simulink model "single_agent_setup"  (R2016a)
settings: Solver=VariableStepAuto  StartTime=0.0  StopTime=400  RelTol=1e-3
model workspace (MAT data in the model file):
  agent_signal = Simulink.Signal
  agent_signal.DataType = 'double'
  agent_signal.Dimensions = 2
  agent_signal.DimensionsMode = 'Variable'
  agent_signal.Complexity = 'real'
  agent_signal.SampleTime = -1
  agent_signal.SamplingMode = 'auto'
libraries: simulink x3, vrlib x3
settings Model: Creator=jcfinnerup  LastModifiedBy=jcfinnerup

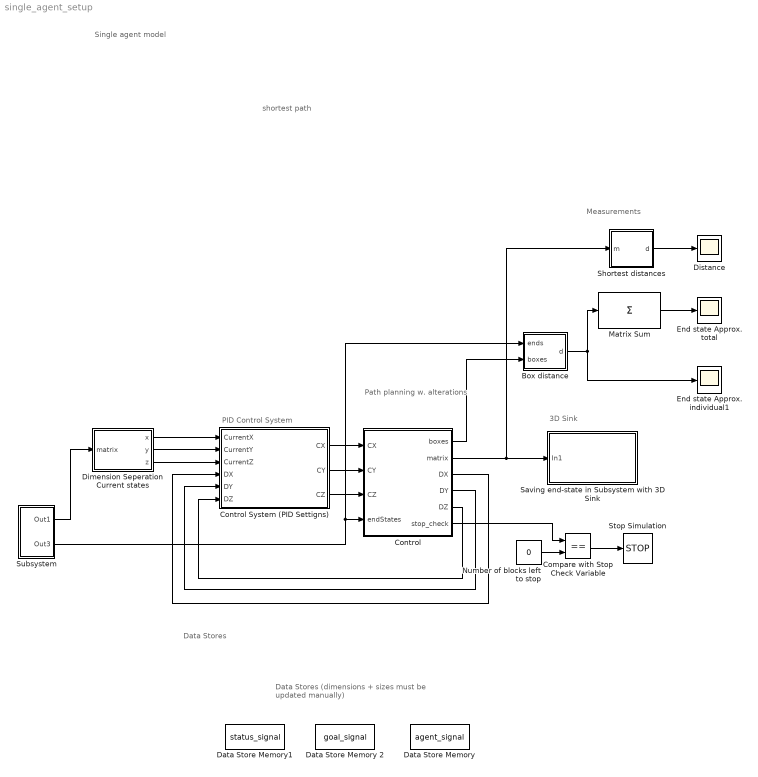
== system single_agent_setup ==
  note: Data Stores
  note: Path planning
      | w.
      | alterations
  note: Single agent model
  note: PID Control System
  note: Data Stores
      | (dimensions + sizes
      | must be updated manually)
  note: 3D Sink
  note: Measurements
  note: shortest path
  Box distance : MATLAB Function  TreatAsAtomicUnit=on
  Compare with Stop Check Variable : RelationalOperator  Operator===  OutDataTypeStr=boolean
  Control : MATLAB Function
  Control System (PID Settigns) : Subsystem
  Data Store Memory : DataStoreMemory  DataStoreName=agent_signal  ReadBeforeWriteMsg=warning  WriteAfterWriteMsg=warning  WriteAfterReadMsg=warning  InitialValue=[-1;-1]  VectorParams1D=off  ShowAdditionalParam=off  OutDataTypeStr=double
  Data Store Memory 2 : DataStoreMemory  DataStoreName=goal_signal  ReadBeforeWriteMsg=warning  WriteAfterWriteMsg=warning  WriteAfterReadMsg=warning  InitialValue=[0, 0, 0, 0, 0, 0, 0, 0, 0]  VectorParams1D=off  ShowAdditionalParam=off  OutDataTypeStr=double
  Data Store Memory1 : DataStoreMemory  DataStoreName=status_signal  ReadBeforeWriteMsg=warning  WriteAfterWriteMsg=warning  WriteAfterReadMsg=warning  InitialValue=[0,0,0,0,0,0,0,0,0;0,0,0,0,0,0,0,0,0]  VectorParams1D=off  ShowAdditionalParam=off  OutDataTypeStr=double
  "Dimension Seperation Current states " : MATLAB Function  TreatAsAtomicUnit=on
  Distance : Scope
  End state Approx. individual1 : Scope
  End state Approx. total : Scope
  Matrix Sum : Sum  Inputs=+
  Number of blocks left to stop : Constant  Value=0
  Saving end-state in Subsystem with 3D Sink : Subsystem
  Shortest distances : MATLAB Function  TreatAsAtomicUnit=on
  Stop Simulation : Stop
  Subsystem : Subsystem
  wires:
  "Dimension Seperation Current states "/1(x) -> Control System (PID Settigns)/1(CurrentX)
  "Dimension Seperation Current states "/2(y) -> Control System (PID Settigns)/2(CurrentY)
  "Dimension Seperation Current states "/3(z) -> Control System (PID Settigns)/3(CurrentZ)
  Control System (PID Settigns)/2(CY) -> Control/2(CY)
  Control System (PID Settigns)/3(CZ) -> Control/3(CZ)
  Control System (PID Settigns)/1(CX) -> Control/1(CX)
  Control/3(DX) -> Control System (PID Settigns)/4(DX)
  Control/4(DY) -> Control System (PID Settigns)/5(DY)
  Control/5(DZ) -> Control System (PID Settigns)/6(DZ)
  Number of blocks left to stop/1 -> Compare with Stop Check Variable/2
  Control/6(stop_check) -> Compare with Stop Check Variable/1
  Compare with Stop Check Variable/1 -> Stop Simulation/1
  Control/2(matrix) -> Shortest distances/1(m), Saving end-state in Subsystem with 3D Sink/1(In1)
  Subsystem/2(Out3) -> Box distance/1(ends), Control/4(endStates)
  Subsystem/1(Out1) -> "Dimension Seperation Current states "/1(matrix)
  Box distance/1(d) -> End state Approx. individual1/1, Matrix Sum/1
  Matrix Sum/1 -> End state Approx. total/1
  Shortest distances/1(d) -> Distance/1
  Control/1(boxes) -> Box distance/2(boxes)

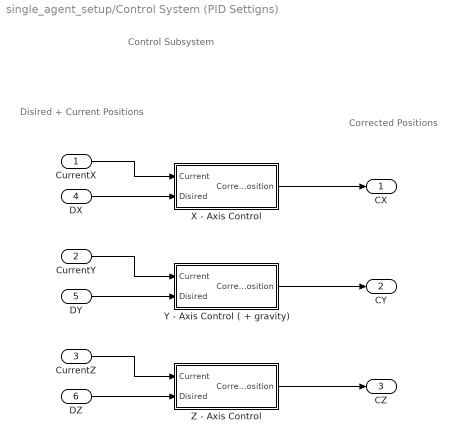
== system single_agent_setup/Control System (PID Settigns) ==
  note: Control Subsystem
  note: Corrected
      | Positions
  note: Disired + Current
      | Positions
  CurrentX : Inport
  CurrentY : Inport  Port=2
  CurrentZ : Inport  Port=3
  DX : Inport  Port=4
  DY : Inport  Port=5
  DZ : Inport  Port=6
  X - Axis Control : Subsystem
  Y - Axis Control ( + gravity) : Subsystem
  "Z - Axis Control " : Subsystem
  CX : Outport
  CY : Outport  Port=2
  CZ : Outport  Port=3
  wires:
  CurrentX/1 -> X - Axis Control/1(Current)
  DX/1 -> X - Axis Control/2(Disired)
  DY/1 -> Y - Axis Control ( + gravity)/2(Disired)
  CurrentY/1 -> Y - Axis Control ( + gravity)/1(Current)
  DZ/1 -> "Z - Axis Control "/2(Disired)
  CurrentZ/1 -> "Z - Axis Control "/1(Current)
  X - Axis Control/1(Corrected Position) -> CX/1
  Y - Axis Control ( + gravity)/1(Corrected Position) -> CY/1
  "Z - Axis Control "/1(Corrected Position) -> CZ/1

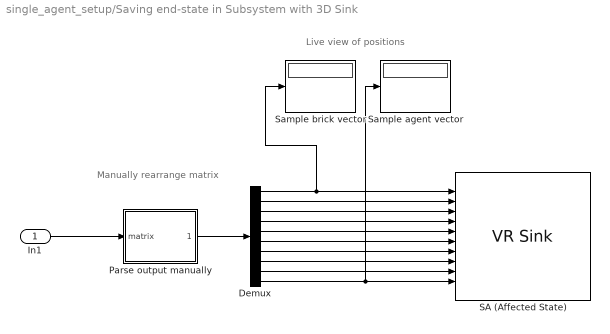
== system single_agent_setup/Saving end-state in Subsystem with 3D Sink ==
  note: Manually rearrange
      | matrix
  note: Live view of positions
  In1 : Inport
  Demux : Demux  Outputs=10
  Parse output manually : MATLAB Function  TreatAsAtomicUnit=on
  "SA (Affected State) " : vrlib/VR Sink  InstantiateOnLoad=on  SampleTime=0.1  ViewEnable=on  RemoteChange=off  RemoteView=off  FieldsWritten=B1.translation.3.1.1.double#B2.translation.3.1.1.double#B3.translation.3.1.1.double#B4.translation.3.1.1.double#B5.translation.3.1.1.double#B6.translation.3.1.1.double#B7.translation.3.1.1.double#B8.translation.3.1.1.double#B9.translation.3.1.1.double#A1.translation.3.1.1.double  WorldFileName=VR3D_SA/single_agent_setup.wrl  WorldDescription=Single Agent Track  AutoView=off  VideoDimensions=[]  AllowVariableSize=off
  Sample agent vector : Display
  "Sample brick vector " : Display
  wires:
  In1/1 -> Parse output manually/1(matrix)
  Demux/10 -> "SA (Affected State) "/10, Sample agent vector/1
  Demux/1 -> "SA (Affected State) "/1, "Sample brick vector "/1
  Parse output manually/1(formatted) -> Demux/1
  Demux/2 -> "SA (Affected State) "/2
  Demux/3 -> "SA (Affected State) "/3
  Demux/4 -> "SA (Affected State) "/4
  Demux/5 -> "SA (Affected State) "/5
  Demux/6 -> "SA (Affected State) "/6
  Demux/7 -> "SA (Affected State) "/7
  Demux/8 -> "SA (Affected State) "/8
  Demux/9 -> "SA (Affected State) "/9

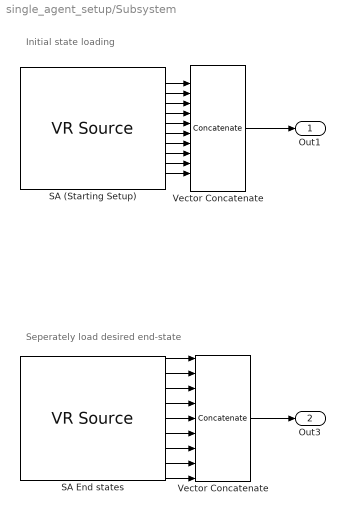
== system single_agent_setup/Subsystem ==
  note: Initial state loading
  note: Seperately load desired end-state
  "SA End states " : vrlib/VR Source  InstantiateOnLoad=on  SampleTime=0.1  ViewEnable=on  RemoteChange=off  RemoteView=off  FieldsRead=E1.translation.1.3.1.double#E2.translation.1.3.1.double#E3.translation.1.3.1.double#E4.translation.1.3.1.double#E5.translation.1.3.1.double#E6.translation.1.3.1.double#E7.translation.1.3.1.double#E8.translation.1.3.1.double#E9.translation.1.3.1.double  WorldFileName=VR3D_SA/single_agent_setup.wrl  WorldDescription=Single Agent Track  AutoView=off  VideoDimensions=[]  AllowVariableSize=off
  SA (Starting Setup) : vrlib/VR Source  InstantiateOnLoad=on  SampleTime=1  ViewEnable=on  RemoteChange=off  RemoteView=off  FieldsRead=B1.translation.1.3.1.double#B2.translation.1.3.1.double#B3.translation.1.3.1.double#B4.translation.1.3.1.double#B5.translation.1.3.1.double#B6.translation.1.3.1.double#B7.translation.1.3.1.double#B8.translation.1.3.1.double#B9.translation.1.3.1.double#A1.translation.1.3.1.double  WorldFileName=VR3D_SA/single_agent_setup.wrl  WorldDescription=Single Agent Track  AutoView=off  VideoDimensions=[]  AllowVariableSize=off
  Vector Concatenate : Concatenate  NumInputs=10  Mode=Multidimensional array  ConcatenateDimension=2
  "Vector Concatenate " : Concatenate  NumInputs=9  Mode=Multidimensional array  ConcatenateDimension=2
  Out1 : Outport
  Out3 : Outport  Port=2
  wires:
  Vector Concatenate/1 -> Out1/1
  "Vector Concatenate "/1 -> Out3/1
  SA (Starting Setup)/1 -> Vector Concatenate/1
  SA (Starting Setup)/2 -> Vector Concatenate/2
  SA (Starting Setup)/3 -> Vector Concatenate/3
  SA (Starting Setup)/4 -> Vector Concatenate/4
  SA (Starting Setup)/5 -> Vector Concatenate/5
  SA (Starting Setup)/6 -> Vector Concatenate/6
  SA (Starting Setup)/7 -> Vector Concatenate/7
  SA (Starting Setup)/8 -> Vector Concatenate/8
  SA (Starting Setup)/9 -> Vector Concatenate/9
  SA (Starting Setup)/10 -> Vector Concatenate/10
  "SA End states "/1 -> "Vector Concatenate "/1
  "SA End states "/2 -> "Vector Concatenate "/2
  "SA End states "/3 -> "Vector Concatenate "/3
  "SA End states "/4 -> "Vector Concatenate "/4
  "SA End states "/5 -> "Vector Concatenate "/5
  "SA End states "/6 -> "Vector Concatenate "/6
  "SA End states "/7 -> "Vector Concatenate "/7
  "SA End states "/8 -> "Vector Concatenate "/8
  "SA End states "/9 -> "Vector Concatenate "/9

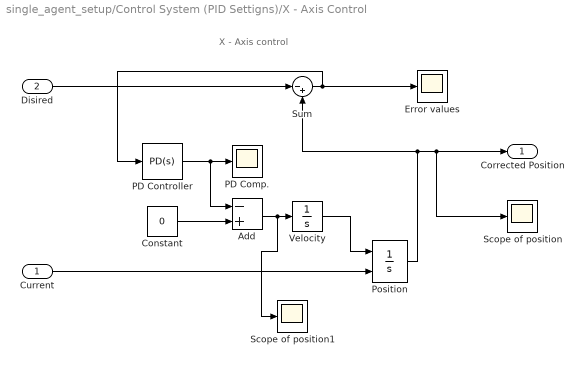
== system single_agent_setup/Control System (PID Settigns)/X - Axis Control ==
  note: X - Axis control
  Current : Inport
  Disired : Inport  Port=2
  Add : Sum  Inputs=-+
  Constant : Constant  Value=0
  Error values : Scope
  "PD Comp. " : Scope
  PD Controller : simulink/Continuous/PID Controller  Controller=PD  TimeDomain=Continuous-time  SampleTime=-1  IntegratorMethod=Forward Euler  FilterMethod=Forward Euler  Form=Ideal  UseFilter=on  ControllerParametersSource=internal  P=0.1  I=5  D=0.1  N=100  InitialConditionSource=internal  InitialConditionForIntegrator=10  InitialConditionForFilter=0  ExternalReset=none  LimitOutput=off  UpperSaturationLimit=1  LowerSaturationLimit=-1  LinearizeAsGain=on  AntiWindupMode=none  Kb=1  TrackingMode=off  Kt=1  PParamMin=[]  PParamMax=[]  IParamMin=[]  IParamMax=[]  DParamMin=[]  DParamMax=[]  NParamMin=[]  NParamMax=[]  KbParamMin=[]  KbParamMax=[]  KtParamMin=[]  KtParamMax=[]  POutMin=[]  POutMax=[]  IOutMin=[]  IOutMax=[]  DOutMin=[]  DOutMax=[]  NOutMin=[]  NOutMax=[]  KbOutMin=[]  KbOutMax=[]  KtOutMin=[]  KtOutMax=[]  IntegratorOutMin=[]  IntegratorOutMax=[]  FilterOutMin=[]  FilterOutMax=[]  SumOutMin=[]  SumOutMax=[]  SumI1OutMin=[]  SumI1OutMax=[]  SumI2OutMin=[]  SumI2OutMax=[]  SumI3OutMin=[]  SumI3OutMax=[]  SumDOutMin=[]  SumDOutMax=[]  SaturationOutMin=[]  SaturationOutMax=[]  IntegratorContinuousStateAttributes=''  IntegratorStateMustResolveToSignalObject=off  IntegratorRTWStateStorageClass=Auto  FilterContinuousStateAttributes=''  FilterStateMustResolveToSignalObject=off  FilterRTWStateStorageClass=Auto  DifferentiatorICPrevScaledInput=0  DifferentiatorOutMin=[]  DifferentiatorOutMax=[]
  Position : Integrator  InitialConditionSource=external  LowerSaturationLimit=0
  Scope of position : Scope
  Scope of position1 : Scope
  Sum : Sum  Inputs=|-+
  Velocity : Integrator  LimitOutput=on  UpperSaturationLimit=15  LowerSaturationLimit=-15
  Corrected Position : Outport
  wires:
  Disired/1 -> Sum/1
  Sum/1 -> Error values/1, PD Controller/1
  PD Controller/1 -> Add/1, "PD Comp. "/1
  Add/1 -> Scope of position1/1, Velocity/1
  Current/1 -> Position/2
  Position/1 -> Sum/2, Scope of position/1, Corrected Position/1
  Velocity/1 -> Position/1
  Constant/1 -> Add/2

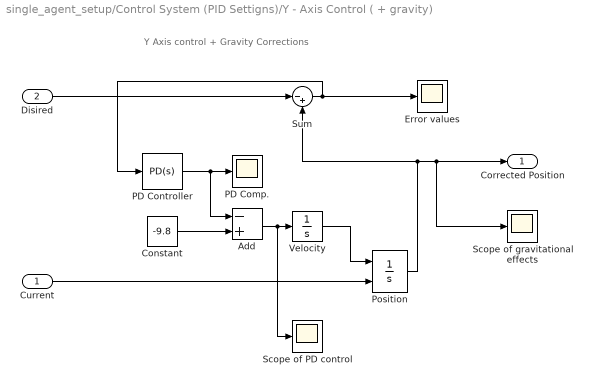
== system single_agent_setup/Control System (PID Settigns)/Y - Axis Control ( + gravity) ==
  note: Y Axis control + Gravity Corrections
  Current : Inport
  Disired : Inport  Port=2
  Add : Sum  Inputs=-+  OutMin=[-9.8]
  Constant : Constant  Value=-9.8
  Error values : Scope
  "PD Comp. " : Scope
  PD Controller : simulink/Continuous/PID Controller  Controller=PD  TimeDomain=Continuous-time  SampleTime=-1  IntegratorMethod=Forward Euler  FilterMethod=Forward Euler  Form=Parallel  UseFilter=on  ControllerParametersSource=internal  P=5  I=1  D=2  N=100  InitialConditionSource=internal  InitialConditionForIntegrator=10  InitialConditionForFilter=0  ExternalReset=none  LimitOutput=on  UpperSaturationLimit=0  LowerSaturationLimit=-50  LinearizeAsGain=off  AntiWindupMode=none  Kb=1  TrackingMode=off  Kt=1  PParamMin=[]  PParamMax=[]  IParamMin=[]  IParamMax=[]  DParamMin=[]  DParamMax=[]  NParamMin=[]  NParamMax=[]  KbParamMin=[]  KbParamMax=[]  KtParamMin=[]  KtParamMax=[]  POutMin=[]  POutMax=[]  IOutMin=[]  IOutMax=[]  DOutMin=[]  DOutMax=[]  NOutMin=[]  NOutMax=[]  KbOutMin=[]  KbOutMax=[]  KtOutMin=[]  KtOutMax=[]  IntegratorOutMin=[]  IntegratorOutMax=[]  FilterOutMin=[]  FilterOutMax=[]  SumOutMin=[]  SumOutMax=[]  SumI1OutMin=[]  SumI1OutMax=[]  SumI2OutMin=[]  SumI2OutMax=[]  SumI3OutMin=[]  SumI3OutMax=[]  SumDOutMin=[]  SumDOutMax=[]  SaturationOutMin=[]  SaturationOutMax=[]  IntegratorContinuousStateAttributes=''  IntegratorStateMustResolveToSignalObject=off  IntegratorRTWStateStorageClass=Auto  FilterContinuousStateAttributes=''  FilterStateMustResolveToSignalObject=off  FilterRTWStateStorageClass=Auto  DifferentiatorICPrevScaledInput=0  DifferentiatorOutMin=[]  DifferentiatorOutMax=[]
  Position : Integrator  InitialConditionSource=external  LimitOutput=on  LowerSaturationLimit=0
  Scope of PD control : Scope
  "Scope of gravitational effects " : Scope
  Sum : Sum  Inputs=|-+
  Velocity : Integrator
  Corrected Position : Outport
  wires:
  Constant/1 -> Add/2
  Velocity/1 -> Position/1
  Position/1 -> Corrected Position/1, "Scope of gravitational effects "/1, Sum/2
  Current/1 -> Position/2
  Add/1 -> Scope of PD control/1, Velocity/1
  PD Controller/1 -> "PD Comp. "/1, Add/1
  Sum/1 -> PD Controller/1, Error values/1
  Disired/1 -> Sum/1

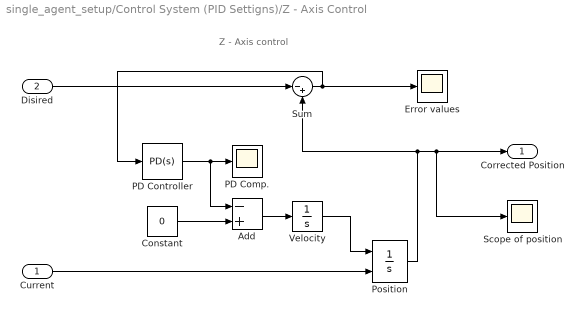
== system single_agent_setup/Control System (PID Settigns)/Z - Axis Control  ==
  note: Z - Axis control
  Current : Inport
  Disired : Inport  Port=2
  Add : Sum  Inputs=-+
  Constant : Constant  Value=0
  Error values : Scope
  "PD Comp. " : Scope
  PD Controller : simulink/Continuous/PID Controller  Controller=PD  TimeDomain=Continuous-time  SampleTime=-1  IntegratorMethod=Forward Euler  FilterMethod=Forward Euler  Form=Ideal  UseFilter=on  ControllerParametersSource=internal  P=2  I=1  D=5  N=100  InitialConditionSource=internal  InitialConditionForIntegrator=10  InitialConditionForFilter=0  ExternalReset=none  LimitOutput=on  UpperSaturationLimit=1  LowerSaturationLimit=-1  LinearizeAsGain=on  AntiWindupMode=none  Kb=1  TrackingMode=off  Kt=1  PParamMin=[]  PParamMax=[]  IParamMin=[]  IParamMax=[]  DParamMin=[]  DParamMax=[]  NParamMin=[]  NParamMax=[]  KbParamMin=[]  KbParamMax=[]  KtParamMin=[]  KtParamMax=[]  POutMin=[]  POutMax=[]  IOutMin=[]  IOutMax=[]  DOutMin=[]  DOutMax=[]  NOutMin=[]  NOutMax=[]  KbOutMin=[]  KbOutMax=[]  KtOutMin=[]  KtOutMax=[]  IntegratorOutMin=[]  IntegratorOutMax=[]  FilterOutMin=[]  FilterOutMax=[]  SumOutMin=[]  SumOutMax=[]  SumI1OutMin=[]  SumI1OutMax=[]  SumI2OutMin=[]  SumI2OutMax=[]  SumI3OutMin=[]  SumI3OutMax=[]  SumDOutMin=[]  SumDOutMax=[]  SaturationOutMin=[]  SaturationOutMax=[]  IntegratorContinuousStateAttributes=''  IntegratorStateMustResolveToSignalObject=off  IntegratorRTWStateStorageClass=Auto  FilterContinuousStateAttributes=''  FilterStateMustResolveToSignalObject=off  FilterRTWStateStorageClass=Auto  DifferentiatorICPrevScaledInput=0  DifferentiatorOutMin=[]  DifferentiatorOutMax=[]
  Position : Integrator  InitialConditionSource=external  LowerSaturationLimit=0
  Scope of position : Scope
  Sum : Sum  Inputs=|-+
  Velocity : Integrator
  Corrected Position : Outport
  wires:
  Constant/1 -> Add/2
  Velocity/1 -> Position/1
  Position/1 -> Corrected Position/1, Scope of position/1, Sum/2
  Current/1 -> Position/2
  Add/1 -> Velocity/1
  PD Controller/1 -> "PD Comp. "/1, Add/1
  Sum/1 -> PD Controller/1, Error values/1
  Disired/1 -> Sum/1

== matlab function single_agent_setup/Box distance ==
  data: ends input; d output; boxes input
function d = dist(ends, boxes)
%#codegen


    distance = zeros(1,length(ends));

    
    for i=1:length(ends)
        this_vec = abs(ends(:,i) - boxes(:,i));
        this_dist = norm(this_vec);
        distance(1, i) = this_dist;
    end
    
d = distance;

== matlab function single_agent_setup/Shortest distances ==
  data: m input; d output
function d = dist(m)
%#codegen


% This function is used to calculate the shortest distance from
% the agents and blocks to other agents or blocks
    
    % Matrix to hold distance
    matrix = m(:,10);
    distance = zeros(1,length(matrix(1,:)));
        
    % Compute Euclidian distance to nearest object
    for i=1:length(matrix(1,:))
        distance(1,i) = 500;
        this_pos = matrix(:,i);
        
        for j=1:length(matrix(1,:))
            % Skip if comparing with self
            if j == i
                continue;
            end
            
            % Calc 3D distance
            this_vec = abs(this_pos - matrix(:,j));
            this_dist = norm(this_vec);
            if distance(1,i) > this_dist
                distance(1,i) = this_dist;
            end
        end
    end
    
d = distance;

== matlab function single_agent_setup/Dimension Seperation Current states  ==
  data: x output; y output; z output; matrix input

function [x,y,z] =  fun(matrix)
    x = matrix(1,:)
    y = matrix(2,:)
    z = matrix(3,:)

== matlab function single_agent_setup/Control ==
  data: boxes output; CX input; CY input; CZ input; endStates input; matrix output; DX output; DY output; DZ output; agent_signal data_store_memory; status_signal data_store_memory; goal_signal data_store_memory; stop_check output
function [boxes, matrix, DX, DY, DZ, stop_check] = fcn(CX, CY, CZ, endStates)
%#codegen

    % Constants 
    block_height = 6;
    block_width = 10;
    agents_at = [10]; % Denotes the indices of the agents
    threshold = 2;
        
    % Variables
    % (Status of box, status of goal)
    % 0: nothing, 1:moving, 2:completed
    global status_signal;
    blocks_moving_to = status_signal;
    
    % (Index of agent, index of end state
    global agent_signal;
    agents_moving_to = agent_signal;
        
    % Assign it not pre-assigned
    if sum(agents_moving_to) == -2
        agents_moving_to = zeros(2,length(agents_at));
        blocks_moving_to = zeros(2,length(endStates));
    end

    
    % Mapping Dimensions of End-States
    EX = endStates(1,:);
    EY = endStates(2,:);
    EZ = endStates(3,:);
    
    % Creating Desired Positions From Current Positions
    DX = CX;
    DY = CY;
    DZ = CZ;
    
    
    
    % Check if simulation is completed
    stop_check = sum(ismember(ismember(blocks_moving_to(2,:), 2),0));
    disp(stop_check);
    
    % Looping through Objects
    % This is the control loop where desired positions are changed
    % Nothing is changed if the agent is already on the way to 
    % the desired position
    % or if the end states are already fulfilled
    
    % Assign an agent to a goal, and a box to an goal
    for a = 1:length(agents_at)
        
        % a = index of agent in agents_moting_to table
        % agent_index = index of agent in all objects
        agent_index = agents_at(a);    
        
%       DY(agent_index) = CY(2)+block_height;
%       DX(agent_index) = CX(2);
%       DZ(agent_index) = CZ(2);
        
        % Check if the agent already has task
        if agents_moving_to(1,a) == 0
            
            % Assign agent to task, with 1
            agents_moving_to(1,a) = 1;
            
            % Check which goal is available
            for i = 1:length(endStates)
                status_of_end_state = ismember(blocks_moving_to(2,i),0);
                if sum(status_of_end_state) == 1
                    
                    % Map goal at index i, with 1 for "moving"
                    blocks_moving_to(2,i) = 1; 
                    
                    % Pick 
                    blocks_moving_to(1,i) = 1;
                    
                    % Reserve agent for box and goal at this index
                    agents_moving_to(2,a) = i;
                    
                    % Break Search for this agent
                    break;
                else
                    % Block is moving 
                end
            end  
        end     
    end
    
    % Assign Desired Positions
    for i = 1:length(agents_at)
        index_of_box_and_goal = agents_moving_to(2,i);
        index_of_agent = agents_at(i);
        
        % Agent Positions
        agent_x = CX(index_of_agent);
        agent_y = CY(index_of_agent);
        agent_z = CZ(index_of_agent);
        agent_pos = [agent_x agent_y agent_z];

        % Assign movement towards box
        if agents_moving_to(1,i) == 1
            
            % Box positions
            box_x = CX(index_of_box_and_goal);
            box_y = CY(index_of_box_and_goal) + block_height;
            box_z = CZ(index_of_box_and_goal);

            % Arrays of these
            box_pos = [box_x box_y box_z];
            
            % Assigning Positions
            DX(index_of_agent) = box_x;
            DY(index_of_agent) = box_y;
            DZ(index_of_agent) = box_z;
            
            % Check if agent is placed correctly
            if sum(abs(box_pos - agent_pos)>threshold) == 0
               disp('Box Reached'); 
               agents_moving_to(1,i) = 2;
            end
        
        % Assign movement towards goal
        elseif agents_moving_to(1,i) == 2;
            % Box positions
            goal_x = EX(index_of_box_and_goal);
            goal_y = EY(index_of_box_and_goal) + block_height;
            goal_z = EZ(index_of_box_and_goal);

            % Arrays of these
            goal_pos = [goal_x goal_y goal_z];  
            
            % Assigning Positions
            DX(index_of_agent) = goal_x;
            DY(index_of_agent) = goal_y;
            DZ(index_of_agent) = goal_z;
            
            CX(index_of_box_and_goal) = agent_x;
            CY(index_of_box_and_goal) = agent_y-(block_height*0.5);
            CZ(index_of_box_and_goal) = agent_z;
            
            % Check if agent is placed correctly
            if sum(abs(goal_pos - agent_pos)>threshold) == 0
               disp('Goal Reached'); 
               agents_moving_to(1, i) = 0;
               blocks_moving_to(1, index_of_box_and_goal) = 2;
               blocks_moving_to(2, index_of_box_and_goal) = 2;
            end
        end
    end
    
    
    % Overwrite physics for boxes for completed goals
    for i = 1:length(blocks_moving_to)    
        if blocks_moving_to(1,i) == 2 % 2 for completed
            CX(i) = EX(i);
            CY(i) = EY(i);
            CZ(i) = EZ(i);
        end
    end
    
    
    
    % Update Global Variables
    agent_signal = agents_moving_to;
    status_signal = blocks_moving_to;

    matrix = [CX;CY;CZ];
    boxes = matrix(1:end,1:end-length(agents_at));

== matlab function single_agent_setup/Saving end-state in Subsystem with 3D Sink/Parse output manually ==
  data: matrix input; formatted output
function formatted = fcn(matrix)
%#codegen

formatted = [
    matrix(:,1)
    matrix(:,2)
    matrix(:,3)
    matrix(:,4)
    matrix(:,5)
    matrix(:,6)
    matrix(:,7)
    matrix(:,8)
    matrix(:,9)
    matrix(:,10)
];
